simulink model "Final_Simulation"  (R2023b)
settings: Solver=FixedStepAuto  StartTime=0.0  StopTime=2  FixedStep=0.001  RelTol=1e-3  AbsTol=1e-3  EnableMultiTasking=on
model workspace (MAT data in the model file):
  Armature_Inductance = 0.001
  Armature_Inductance_NEW = 1.12039737344e-06
  Armature_Inductance_n = 0.00994620821305
  Coulomb_Friction_Force = 1
  Coulomb_Friction_Force_N = 0.0521332457902
  Coulomb_Friction_Force_NEW = 1.64621921379
  Damping_coefficient = 1
  Damping_coefficient_N = 38.8460996806
  Damping_coefficient_NEW = 1.71815570054
  Et = 0.108547063034
  Friction_Force = 1
  Friction_Force_N = 1.46192424023
  Friction_Force_NEW = 2.69201475613
  Friction_coeffient = 0.1
  Friction_coeffient_N = 0.973219921945
  Friction_coeffient_NEW = 354.482161898
  R = 0.962194376059
  Rated_speed = 195.095180091
  Rotor_damping = 1
  Stall_torque = 0.129665131132
  Test_Signals = Simulink.SimulationData.Dataset
  Test_Signals.any.Name = 'Test Signals'
  Test_Signals.any.Version = 3
  Test_Signals.any.Storage = Simulink.SimulationData.Storage.RamDatasetStorage
  Test_Signals.any.Storage.any.Version = 2
  Test_Signals.any.Storage.any.Elements{1} = timeseries
  Test_Signals.any.Storage.any.Elements{1}.Name = 'Estimation'
  Test_Signals.any.Storage.any.Elements{1}.DataInfo = tsdata.datametadata
  Test_Signals.any.Storage.any.Elements{1}.DataInfo.Interpolation = tsdata.interpolation
  Test_Signals.any.Storage.any.Elements{1}.DataInfo.Interpolation.Fhandle : function handle (value not decoded)
  Test_Signals.any.Storage.any.Elements{1}.DataInfo.Interpolation.Name = 'linear'
  Test_Signals.any.Storage.any.Elements{1}.TimeInfo = tsdata.timemetadata
  Test_Signals.any.Storage.any.Elements{1}.TimeInfo.Length = 40
  Test_Signals.any.Storage.any.Elements{1}.TimeInfo.DuplicateTimes = 1
  Test_Signals.any.Storage.any.Elements{1}.TimeInfo.Time_ = [0; 0.25; 0.25; 0.5; 0.5; 0.75; 0.75; 1; 1; 1.25; 1.25; 1.5; 1.5; 1.75; 1.75; 2; 2; 2.25; 2.25; 2.5; 2.5; 2.75; 2.75; 3; 3; 3.25; 3.25; 3.5; 3.5; 3.75; 3.75; 4; 4; 4.25; 4.25; 4.5; 4.5; 4.75; 4.75; 5]
  Test_Signals.any.Storage.any.Elements{1}.TimeInfo.Initialized = 1
  Test_Signals.any.Storage.any.Elements{1}.QualityInfo = tsdata.qualmetadata
  Test_Signals.any.Storage.any.Elements{1}.Data_ = [1; 1; -1; -1; 1; 1; -1; -1; 1; 1; -1; -1; 1; 1; -1; -1; 1; 1; -1; -1; 1; 1; -1; -1; 1; 1; -1; -1; 1; 1; -1; -1; 1; 1; -1; -1; 1; 1; -1; -1]
  Test_Signals.any.Storage.any.Elements{2} = timeseries
  Test_Signals.any.Storage.any.Elements{2}.Name = 'Validation'
  Test_Signals.any.Storage.any.Elements{2}.DataInfo = tsdata.datametadata
  Test_Signals.any.Storage.any.Elements{2}.DataInfo.Interpolation = tsdata.interpolation
  Test_Signals.any.Storage.any.Elements{2}.DataInfo.Interpolation.Fhandle : function handle (value not decoded)
  Test_Signals.any.Storage.any.Elements{2}.DataInfo.Interpolation.Name = 'linear'
  Test_Signals.any.Storage.any.Elements{2}.TimeInfo = tsdata.timemetadata
  Test_Signals.any.Storage.any.Elements{2}.TimeInfo.Length = 10
  Test_Signals.any.Storage.any.Elements{2}.TimeInfo.DuplicateTimes = 1
  Test_Signals.any.Storage.any.Elements{2}.TimeInfo.Time_ = [0; 0.75; 0.75; 1; 1; 1.5; 1.5; 1.75; 1.75; 5]
  Test_Signals.any.Storage.any.Elements{2}.TimeInfo.Initialized = 1
  Test_Signals.any.Storage.any.Elements{2}.QualityInfo = tsdata.qualmetadata
  Test_Signals.any.Storage.any.Elements{2}.Data_ = [0; 0; 1; 1; -1; -1; 1; 1; 0; 0]
  Var = 0
  Var1 = 5
  inertia = 1
  inertia_NEW = 0.00233565531733
  inertia_n = 0.000234701107851
  mechanical_power = 0.00219878017021
  mechanical_power_NEW = 0.60626924632
  xInitial = 1
undefined symbols (not defined in the file): In
libraries: fl_lib x7, ee_lib x3, nesl_utility x3
CloseFcn:
  | try,close(h1_PWMControlledDCMotor),end
  | clear h1_PWMControlledDCMotor
  | 
  | clear simlog_PWMControlledDCMotor
  | clear logsout_PWMControlledDCMotor
  | clear RPM RPM1 tout
Description:
  | PWM-Controlled DC Motor
settings Model: ExtModeTrigDuration=2  Creator=The MathWorks, Inc.  LastModifiedBy=Taha
settings SolverCC: AutoScaleAbsTol=off  AlgebraicLoopSolver=TrustRegion
settings DataIOCC: ExternalInput=PWM_Input_225_PWM.getElement('PWM_Signal')  LimitDataPoints=on  MaxDataPoints=10000  LoadExternalInput=on  SaveFormat=Array  ReturnWorkspaceOutputs=off  SignalLoggingName=logsout_PWMControlledDCMotor
settings OptimizationCC: EnhancedBackFolding=on  PassReuseOutputArgsAs=Individual arguments  ExpressionDepthLimit=2147483647  ZeroExternalMemoryAtStartup=off  ZeroInternalMemoryAtStartup=off  InitFltsAndDblsToZero=on  MaxStackSize=64  OptimizeBlockOrder=speed  DifferentSizesBufferReuse=on  OptimizationCustomize=off  EfficientTunableParamExpr=on
settings DebuggingCC: UnderspecifiedInitializationDetection=Classic  MergeDetectMultiDrivingBlocksExec=none  ParameterTunabilityLossMsg=error  FcnCallInpInsideContextMsg=warning  UnconnectedInputMsg=warning  UnconnectedOutputMsg=warning  UnconnectedLineMsg=warning  StateNameClashWarn=warning  SFUnexpectedBacktrackingDiag=warning  SFNoUnconditionalDefaultTransitionDiag=warning  SFExecutionAtInitializationDiag=none  ArithmeticOperatorsInVariantConditions=warning
settings HardwareCC: ProdBitPerInt=16  ProdBitPerPointer=16  ProdBitPerSizeT=16  ProdBitPerPtrDiffT=16  ProdLargestAtomicFloat=None  ProdWordSize=8  ProdHWDeviceType=Atmel->AVR  UseEmbeddedCoderFeatures=off  UseSimulinkCoderFeatures=off
settings ModelReferenceCC: EnableRefExpFcnMdlSchedulingChecks=on  PropagateSignalLabelsOutOfModel=off
settings SFSimCC: SimUseLocalCustomCode=off  MATLABDynamicMemAlloc=off  CustomCodeUndefinedFunction=UseInterfaceOnly
settings RTWCC: Description=Embedded Coder  SystemTargetFile=ert.tlc  HardwareBoard=Arduino Uno  TemplateMakefile=ert_default_tmf  RTWUseLocalCustomCode=off  Toolchain=Arduino AVR  BuildConfiguration=Faster Runs  DLArmComputeVersion=19.05
settings CodeAppCC: ForceParamTrailComments=on  IgnoreCustomStorageClasses=off  OperatorAnnotations=on  SimulinkDataObjDesc=on  SFDataObjDesc=on  InsertBlockDesc=on
settings ERTTargetCC: SupportContinuousTime=on  SupportNonInlinedSFcns=on  SupportVariableSizeSignals=on  ExtModeTransport=3  ExtModeStaticAlloc=on  ExtModeAutomaticAllocSize=off  ExtModeStaticAllocSize=250  ExtModeMexFile=ext_xcp  ExtModeIntrfLevel=Level2 - Open
settings ConfigComp: CovMetricSettings=dw  CovSaveCumulativeToWorkspaceVar=on  CovSaveSingleToWorkspaceVar=on  CovExternalEMLEnable=off  CovSFcnEnable=off
settings SimscapeCC: SimscapeLogType=all  SimscapeLogSimulationStatistics=on  SimscapeLogName=simlog_PWMControlledDCMotor  SimscapeLogDataHistory=10000

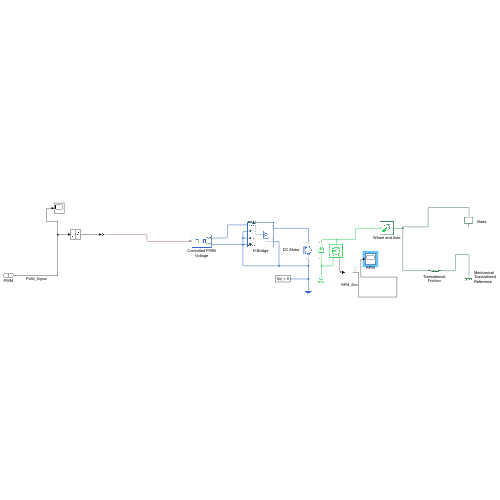
[thumbnail: Simulink's stored preview of the top-level diagram]
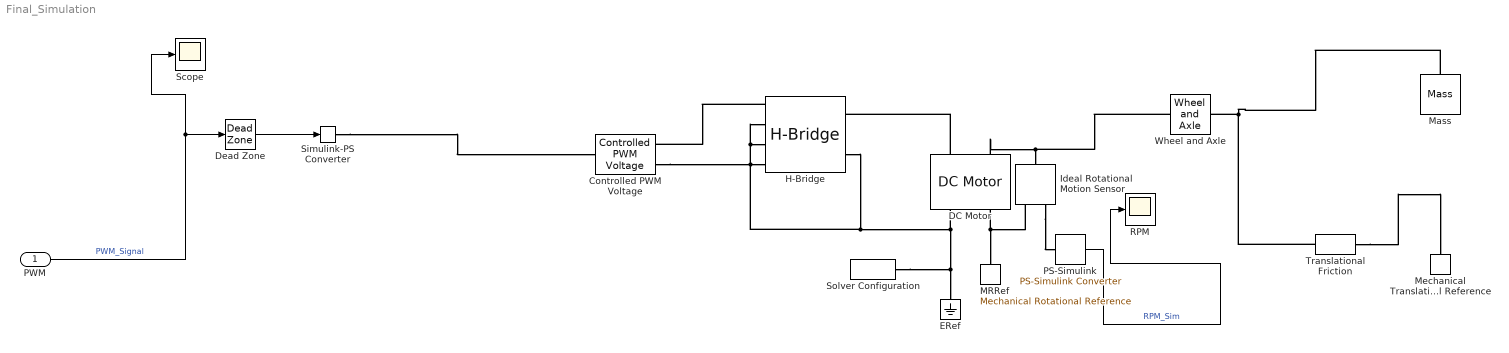
== system Final_Simulation ==
  PWM : Inport
  Controlled PWM Voltage : ee_lib/Integrated Circuits/Controlled PWM Voltage  F=2000 Hz  TD=0 s  pulse_width_offset=0 s  pulse_min=0 s  pwm_or_av=ee.enum.pwm_or_av.averaged  event_type=1  sample_time=5e-6 s  Vmin=0 V  Vmax=5 V  Vm=5 V  u_min=0  u_max=144
      settings: InternalSimscapePortConfiguration="{\"Bottom\":[],\"Left\":[{\"id\":\"u\",\"label\":\"u\",\"type\":\"input\"}],\"Right\":[{\"id\":\"p2\",\"label\":\"PWM\",\"type\":\"foundation.electrical.electrical\"},{\"id\":\"n2\",\"label\":\"REF\",\"type\":\"foundation.electrical.electrical\"}],\"Top\":[]}"
  DC Motor : ee_lib/Electromechanical/Brushed Motors/DC Motor  field_option=ee.enum.field_option.pm  Rf=100 Ohm  Lf=1 H  Laf=0.15 H  If0=0 A  parameterization=ee.enum.dcparam_option.circuit_param  Ra=Ra Ohm  La=I H  emf_or_torque=ee.enum.emf_or_torque.kv  Kv=Eb2 V/(rad/s)  Ki=6.876e-04 N*m/A  T_stall=Stall_torque N*m  w_max=250 rpm  w_rated=Rated_speed rpm  P_rated=mechanical_power_NEW W  V_rated=12 V  lam_param=1  i_noload=0 A  V_i_noload=1.5 V  J=In kg*m^2  lam=RD N*m/(rad/s)  speed0=0 rpm  enable_fault_armature=simscape.enum.onoff.off  rev_faulted=1 / 3  G_faulted_armature=1e-5 S  fault_trigger_armature=ee.enum.faults.faultTrigger.temporal  t_fault_armature=1 s  max_permissible_current_armature=inf A  t_fail_on_current_armature=1 s  enable_fault_field=simscape.enum.onoff.off  G_faulted_field=1e-5 S  fault_trigger_field=ee.enum.faults.faultTrigger.temporal  t_fault_field=1 s  max_permissible_current_field=inf A  t_fail_on_current_field=1 s  fault_action=simscape.enum.assert.action.none  alpha=3.93e-3 1/K  Tmeas=25 degC  thermal_mass=100 J/K  initial_temperature=25 degC
  Dead Zone : DeadZone  LowerValue=0  UpperValue=111
  ERef : fl_lib/Electrical/Electrical Elements/Electrical Reference
  H-Bridge : ee_lib/Semiconductors & Converters/Converters/H-Bridge  supply_ports=ee.enum.supply_ports.hidesupply  pwm_or_av=2  regenerative_braking_mode=2  discontinuous=0  freewheeling_mode=1  Rload=3.38+0.1 Ohm  Lload=1e-5 H  F=4 kHz  Venable=2.5 V  Vmax=5 V  Vreverse=2.5 V  Vbrake=2.5 V  Vm=12 V  Ron=0.1 Ohm  Don=0.1 Ohm  Goff=1e-6 S  Tmeas=298.15 K  Ron2=0.1 Ohm  Don2=0.05 Ohm  Tmeas2=398.15 K  thermal_mass=100 J/K  initial_temperature=298.15 K
  Ideal Rotational Motion Sensor : fl_lib/Mechanical/Mechanical Sensors/Ideal Rotational Motion Sensor  reference=foundation.enum.MeasurementReference.difference  acceleration_port=false  velocity_port=true  position_port=false  wrap_angle=simscape.enum.onoff.off  offset=0 deg
      settings: InternalSimscapePortConfiguration="{\"Bottom\":[],\"Left\":[{\"id\":\"R\",\"label\":\"R\",\"type\":\"foundation.mechanical.rotational.rotational\"}],\"Right\":[{\"id\":\"C\",\"label\":\"C\",\"type\":\"foundation.mechanical.rotational.rotational\"},{\"id\":\"W\",\"label\":\"W\",\"type\":\"output\"}],\"Top\":[]}"
  MRRef : fl_lib/Mechanical/Rotational Elements/Mechanical Rotational Reference
  Mass : fl_lib/Mechanical/Translational Elements/Mass  mass=0.107 kg  num_ports=foundation.enum.numPorts2.one  v_specify=off  v_priority=High  v=0 m/s  v_nominal_specify=off  v_nominal_unit=m/s  v_nominal_value=1  f_specify=off  f_priority=None  f=0 N  f_nominal_specify=off  f_nominal_unit=N  f_nominal_value=1
  Mechanical Translational Reference : fl_lib/Mechanical/Translational Elements/Mechanical Translational Reference
  PS-Simulink : nesl_utility/PS-Simulink Converter  PhysicalDomain=network_engine_domain  SubClassName=ps_output  LeftPortType=input  RightPortType=output  PseudoPeriodic=off  Frequencies=[]  VectorFormat=1-D array  Unit=rpm  AffineConversion=off
  RPM : Scope
  Scope : Scope
  Simulink-PS Converter : nesl_utility/Simulink-PS Converter  PhysicalDomain=network_engine_domain  SubClassName=ps_input  LeftPortType=input  RightPortType=output  PseudoPeriodic=off  Frequencies=[]  NoiseDistribution=none  NoiseParameters=[]  Unit=1  AffineConversion=off  FilteringAndDerivatives=provide  SimscapeFilterOrder=1  InputFilterTimeConstant=0.001  UdotUserProvided=0
  Solver Configuration : nesl_utility/Solver Configuration  PhysicalDomain=network_engine_domain  SubClassName=solver  LeftPortType=input  RightPortType=generic  Tones=[]  Harmonics=[]  SimulateNoise=off  Profile=off  UseLocalSampling=off  EnableSwitchedLinearOptims=on  FrequencyDomain=off  UseCCode=off  RelTol=0.001  AbsTol=1e-06  MinStep=1e-09  ToWorkspace=off  RevertToSquareIcSolve=off  NumHomotopyIterations=100  PhasorMode=off  PhasorModeNumHarmonics=1  ConsistencySolver=NEWTON_FTOL  IndexReductionMethod=DerivativeReplacement  DoDC=off  ResidualTolerance=1e-9  ConsistencyTolSource=GLOBAL  ConsistencyAbsTol=0.001  ConsistencyRelTol=0.001  ConsistencyTolFactor=0.001  UseLocalSolver=off  LocalSolverChoice=NE_BACKWARD_EULER_ADVANCER  ResolveIndetEquations=on  FunctionEvalNumThread=1  LocalSolverSampleTime=5e-6  DoFixedCost=off  MaxNonlinIter=4  MaxModeIter=2  ComputeImpulses=off  ImpulseIterations=2  LinearAlgebra=auto  LinearAlgebraNumThread=0  EquationFormulation=NE_TIME_EF  DelaysMemoryBudget=1024  AutomaticFiltering=on  FilteringTimeConstant=0.001  PartitionStorageMethod=AS_NEEDED  PartitionMemoryBudget=1024  PartitionMethod=FAST  MultibodyUseLocalSolver=off  MultibodyLocalSolverChoice=ODE1  MultibodyLocalSolverSampleTime=0.001
  Translational Friction : fl_lib/Mechanical/Translational Elements/Translational Friction  brkwy_frc=FF2 N  brkwy_vel=V m/s  Col_frc=FF2 N  visc_coef=VFC N*s/m  v_specify=off  v_priority=None  v=0 m/s  v_nominal_specify=off  v_nominal_unit=m/s  v_nominal_value=1  f_specify=off  f_priority=None  f=0 N  f_nominal_specify=off  f_nominal_unit=N  f_nominal_value=1
      settings: InternalSimscapePortConfiguration="{\"Bottom\":[],\"Left\":[{\"id\":\"R\",\"label\":\"R\",\"type\":\"foundation.mechanical.translational.translational\"}],\"Right\":[{\"id\":\"C\",\"label\":\"C\",\"type\":\"foundation.mechanical.translational.translational\"}],\"Top\":[]}"
  Wheel and Axle : fl_lib/Mechanical/Mechanisms/Wheel and Axle  R=1.1 cm  or=1  t_specify=off  t_priority=None  t=0 N*m  t_nominal_specify=off  t_nominal_unit=N*m  t_nominal_value=1  f_specify=off  f_priority=None  f=0 N  f_nominal_specify=off  f_nominal_unit=N  f_nominal_value=1
  wires:
  PS-Simulink/1 -> RPM/1  "RPM_Sim"
  PWM/1 -> Scope/1, Dead Zone/1  "PWM_Signal"
  Dead Zone/1 -> Simulink-PS Converter/1
  connections:
  DC Motor/LConn1 -- H-Bridge/RConn1
  Translational Friction/RConn1 -- Mechanical Translational Reference/LConn1
  Ideal Rotational Motion Sensor/RConn1 -- MRRef/LConn1 -- DC Motor/RConn2
  H-Bridge/RConn2 -- Controlled PWM Voltage/RConn2 -- H-Bridge/LConn2 -- H-Bridge/LConn3 -- H-Bridge/LConn4 -- ERef/LConn1 -- Solver Configuration/RConn1 -- DC Motor/RConn1
  Translational Friction/LConn1 -- Mass/LConn1 -- Wheel and Axle/RConn1
  Wheel and Axle/LConn1 -- DC Motor/LConn2 -- Ideal Rotational Motion Sensor/LConn1
  Ideal Rotational Motion Sensor/RConn2 -- PS-Simulink/LConn1
  H-Bridge/LConn1 -- Controlled PWM Voltage/RConn1
  Simulink-PS Converter/RConn1 -- Controlled PWM Voltage/LConn1
